simulink model "SanctuaryFarmSystem"  (R2021a)
settings: Solver=FixedStepDiscrete  StartTime=0  StopTime=24  FixedStep=1e-06  MaxStep=0.0001  RelTol=1e-6
undefined symbols (not defined in the file): Acid, C, DCDCsampletime, f_sw, L, Lead, sample_time_powergui
libraries: spsVoltageMeasurementLib x4, spsCurrentMeasurementLib x2, spsSeriesRLCBranchLib x2, spsBatteryLib x1, spsDiodeLib x1, spsGroundLib x1, spsMosfetLib x1, spsPVArrayLib x1, simulink x1, spsPWMGeneratorDCDCLib x1, spspowerguiLib x1
settings Model: SimulationMode=accelerator  PacingRate=0.025000  Creator=mike  LastModifiedBy=mike
settings SolverCC: InitialStep=0.0001
settings GRTTargetCC: RTWCAPISignals=on  RTWCAPIParams=on

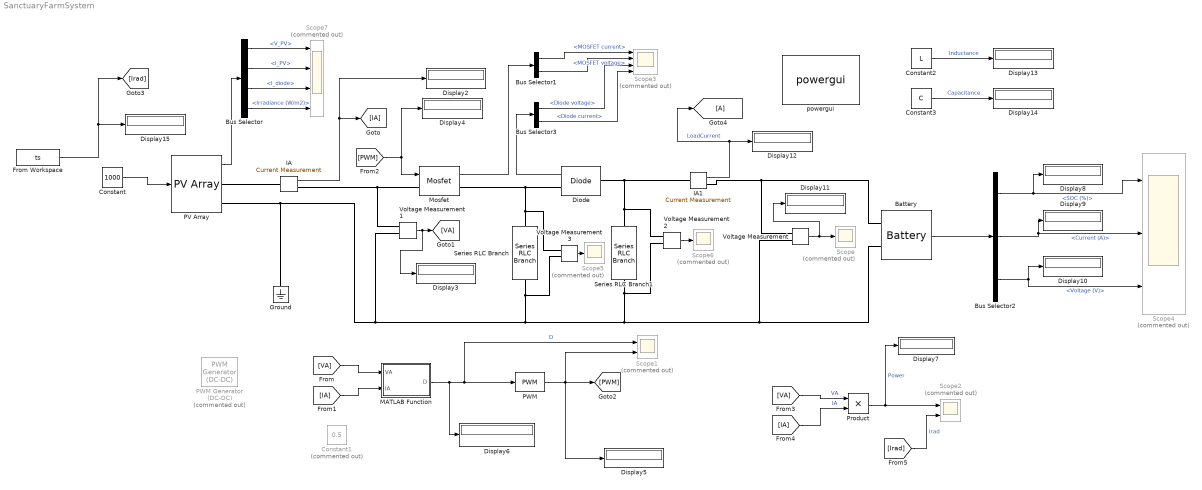
== system SanctuaryFarmSystem ==
  Battery : spsBatteryLib/Battery  BatType=Lead-Acid  ShowTempParam=off  ThermalPreset=no  ShowAgeParam=off  NomV=48  NomQ=200  SOC=50  Batt_Tr=5  PresetModel=on  MaxQ=208.3333  MinV=36  FullV=52.2632  Dis_rate=40  R=0.0024  Normal_OP=62.0556  expZone="[48.8684     0.666667]"  current=[6.5 13 32.5]  Units=Time  Tci=20  NomT=20  T2=-30  MaxQ2=4.8  FullV2=7.1  Normal_OP2=5.655  expZone2="[6.58           1]"  Rca=0.6  ti=2000  Dp=0  Neq0=0  Tsim=1e6  Ta1=25  Qeol=5.4*0.9  Reol=0.013333*1.2  Char_age=[2.3478, 3]  Dis_age=[2.3478, 10]  N1=1500  N2=10500  N3=1000  N4=1400  Ta2=45  N5=950
  Bus Selector : BusSelector  OutputSignals=V_PV,I_PV,I_diode,Irradiance (W/m2)
  Bus Selector1 : BusSelector  OutputSignals=MOSFET current,MOSFET voltage
  Bus Selector2 : BusSelector  OutputSignals=SOC (%),Current (A),Voltage (V)
  Bus Selector3 : BusSelector  OutputSignals=Diode voltage,Diode current
  Constant : Constant  Value=1000
  Constant1 : Constant  Commented=on  Value=0.5
  Constant2 : Constant  Value=L
  Constant3 : Constant  Value=C
  Diode : spsDiodeLib/Diode  Ron=0.001  Lon=0  Vf=0.8  IC=0  UseSnubber=0  Rs=500  Cs=250e-9  Measurements=on
  Display{2..15} (14 alike) : Display
  From Workspace : FromWorkspace  VariableName=ts
  Ground : spsGroundLib/Ground  LConnTagsString=a
  IA : spsCurrentMeasurementLib/Current Measurement  PhasorSimulation=off  OutputType=Complex  PSBequivalent=0
  IA1 : spsCurrentMeasurementLib/Current Measurement  PhasorSimulation=off  OutputType=Complex  PSBequivalent=0
  MATLAB Function : MATLAB Function  TreatAsAtomicUnit=on
  Mosfet : spsMosfetLib/Mosfet  Ron=0.1  Lon=0  Rd=0.01  Vfd=0  IC=0  Rs=1e5  Cs=inf  Measurements=on
  PV Array : spsPVArrayLib/PV Array  Npar=2  Nser=1  PlotType=one module @ 25 deg.C & specified irradiances  S_vec=[1000 500 100]  Temp_C_vec="[ 45 25  ]"  ModuleName=User-defined  PlotWhenSelected=off  Pm=550.2267  Ncell=144  Voc=49.95  Isc=14.05  Vm=41.97  Im=13.11  beta_Voc_pc=-0.35  alpha_Isc_pc=0.05  beta_Voc=-0.17482  alpha_Isc=0.007025  IL=14.063  I0=3.2435e-10  nI=0.55179  Rsh=145.0403  Rs=0.13419  RobustModel=on  RobustCellTemperature=25  BAL=on  Tc=1e-6  Tfilter=5e-5
  PWM : simulink/Discontinuities/PWM  DisableCoverage=on  Period=1/f_sw  DisallowZeroDutyCycle=off  RunAtFixedTimeIntervals=on  SampleTime=DCDCsampletime
  PWM Generator (DC-DC) : spsPWMGeneratorDCDCLib/PWM Generator (DC-DC)  Commented=on  Fsw=f_sw  Ts=DCDCsampletime
  Product : Product
  Scope : Scope  Commented=on
  Scope1 : Scope  Commented=on  NumInputPorts=2
  Scope2 : Scope  Commented=on  NumInputPorts=2
  Scope3 : Scope  Commented=on  NumInputPorts=4
  Scope4 : Scope  Commented=on  NumInputPorts=3
  Scope5 : Scope  Commented=on
  Scope6 : Scope  Commented=on
  Scope7 : Scope  Commented=on  NumInputPorts=4
  Series RLC Branch : spsSeriesRLCBranchLib/Series RLC Branch  LConnTagsString=__new0  RConnTagsString=__new0  BranchType=L  Resistance=1  Inductance=L  SetiL0=off  InitialCurrent=0  Capacitance=1e-6  Setx0=off  InitialVoltage=0  Measurements=Branch voltage and current
  Series RLC Branch1 : spsSeriesRLCBranchLib/Series RLC Branch  LConnTagsString=__new0  RConnTagsString=__new0  BranchType=C  Resistance=1  Inductance=1e-3  SetiL0=off  InitialCurrent=0  Capacitance=C  Setx0=off  InitialVoltage=0  Measurements=Branch voltage and current
  Voltage Measurement{,1..3} (4 alike) : spsVoltageMeasurementLib/Voltage Measurement  PhasorSimulation=off  OutputType=Complex  PSBequivalent=0
  powergui : spspowerguiLib/powergui  Priority=1  SimulationMode=Discrete  SampleTime=sample_time_powergui  frequency=60  Iterations=50  frequencyindice=0  Pbase=100e6  ErrMax=1e-4  UnitsV=kV  UnitsW=MW  buscounter=0  FunctionMessages=off  echomessages=off  EnableUseOfTLC=off  CurrentSourceSwitches=off  DisableSnubberDevices=off  DisableRonSwitches=off  DisableVfSwitches=off  DisplayEquations=on  AutomaticDiscreteSolvers=on  SolverType=Tustin/Backward Euler (TBE)  Interpol=off  ExternalGateDelay=off  methode=off  Ts=100  x0status=zero  SPID=on  SwTol=0  HookPort=off  NonlinearTolerance=1e-4  nMaxIteration=10000  ContinueOnMaxIteration=on  RestoreLinks=warning  ResistiveCurrentMeasurement=off  Frange=[0:2:500]  Ylog=off  Xlog=on  ShowGrid=off  save=off  variable=ZData  structure=0  ZoomFFT=off  StartTime=0.0  cycles=1  DisplayStyle=1  fundamental=60  FreqAxis=off  MaxFrequency=1000  frequencyindicesteady=1  RmsSteady=1  display=off
  wires:
  Voltage Measurement/1 -> Display11/1, Scope/1
  IA/1 -> [IA], Display2/1
  Voltage Measurement1/1 -> Display3/1, [VA]
  [VA] -> MATLAB Function/1(VA)
  [IA] -> MATLAB Function/2(IA)
  MATLAB Function/1(D) -> Display6/1, PWM/1, Scope1/1  "D"
  PWM/1 -> Scope1/2, Display5/1, [PWM]
  [PWM] -> Display4/1, Mosfet/1
  [VA] -> Product/1  "VA"
  [IA] -> Product/2  "IA"
  Product/1 -> Display7/1, Scope2/1  "Power"
  Mosfet/1 -> Bus Selector1/1
  Battery/1 -> Bus Selector2/1
  Bus Selector2/2 -> Display9/1, Scope4/2  "<Current (A)>"
  Bus Selector2/1 -> Display8/1, Scope4/1  "<SOC (%)>"
  IA1/1 -> Display12/1, [A]  "LoadCurrent"
  Constant2/1 -> Display13/1  "Inductance"
  Constant3/1 -> Display14/1  "Capacitance"
  From Workspace/1 -> Display15/1, [Irad]
  Voltage Measurement3/1 -> Scope5/1
  Voltage Measurement2/1 -> Scope6/1
  [Irad] -> Scope2/2  "Irad"
  PV Array/1 -> Bus Selector/1
  Bus Selector/1 -> Scope7/1  "<V_PV>"
  Bus Selector/2 -> Scope7/2  "<I_PV>"
  Bus Selector/3 -> Scope7/3  "<I_diode>"
  Bus Selector/4 -> Scope7/4  "<Irradiance (W/m2)>"
  Bus Selector1/1 -> Scope3/1  "<MOSFET current>"
  Bus Selector1/2 -> Scope3/2  "<MOSFET voltage>"
  Bus Selector2/3 -> Scope4/3, Display10/1  "<Voltage (V)>"
  Diode/1 -> Bus Selector3/1
  Bus Selector3/1 -> Scope3/3  "<Diode voltage>"
  Bus Selector3/2 -> Scope3/4  "<Diode current>"
  Constant/1 -> PV Array/1
  connections:
  Mosfet/RConn1 -- Voltage Measurement3/LConn1 -- Series RLC Branch/LConn1 -- Diode/RConn1
  Series RLC Branch1/LConn1 -- Voltage Measurement2/LConn1 -- IA1/LConn1 -- Diode/LConn1
  Series RLC Branch1/RConn1 -- Voltage Measurement2/LConn2 -- Voltage Measurement3/LConn2 -- Series RLC Branch/RConn1 -- Ground/LConn1 -- PV Array/RConn2 -- Voltage Measurement1/LConn2 -- Voltage Measurement/LConn1 -- Battery/LConn1
  IA/RConn1 -- Voltage Measurement1/LConn1 -- Mosfet/LConn1
  PV Array/RConn1 -- IA/LConn1
  Voltage Measurement/LConn2 -- IA1/RConn1 -- Battery/LConn2

== matlab function SanctuaryFarmSystem/MATLAB Function ==
  data: VA input; D output; IA input
function D = fcn(VA, IA)

persistent VAprev
persistent PAprev
persistent Dprev

changeBy = 0.0001;

if isempty(VAprev)
    VAprev = 0;
end

if isempty(PAprev)
    PAprev = 0;
end

if isempty(Dprev)
    Dprev = 0.5;
end

D = Dprev;
PA = VA*IA;
DeltaVA = VA-VAprev;
DeltaPA = PA-PAprev;

if DeltaPA>0
    if DeltaVA>0
        D=Dprev-changeBy;
    elseif DeltaVA<0
        D=Dprev+changeBy;
    end
elseif DeltaPA<0
    if DeltaVA>0
        D=Dprev+changeBy;
    elseif DeltaVA<0
        D=Dprev-0.001;
    end
end

VAprev = VA;
PAprev = PA;
Dprev = D;


%Max and Min MPPT duty cycle
if D>0.9
    D=0.9;
elseif D<0
    D=0;
end
